simulink model "KitGewerk2_v1_2_Kommunikation_robi"  (R2014a)
settings: Solver=ode3  StartTime=0.0  StopTime=inf  FixedStep=0.005  RelTol=1e-3
undefined symbols (not defined in the file or in its folder): Com1, Com2, none
libraries: slrtlib x14, dspswit3 x3, simulink x2, xpcseriallib x2
(part 1 of 2)
CloseFcn:
  | rtwprivate ssgencode ModelCloseRequest Robotino_Strecke_reall_2009
settings Model: SimulationMode=external  BufferReuse=off  Creator=atlabor  LastModifiedBy=atlabor
settings SolverCC: EnableConcurrentExecution=on
settings DataIOCC: LimitDataPoints=off  SignalLoggingSaveFormat=ModelDataLogs
settings OptimizationCC: BlockReduction=off  OptimizeBlockIOStorage=off  BufferReuse=off  GlobalBufferReuse=off  ExpressionFolding=off  ExpressionDepthLimit=2147483647  LocalBlockOutputs=off  InitFltsAndDblsToZero=on
settings DebuggingCC: SaveWithParameterizedLinksMsg=none  UnderspecifiedInitializationDetection=Classic  FcnCallInpInsideContextMsg=UseLocalSettings  StateNameClashWarn=warning
settings HardwareCC: ProdIntDivRoundTo=Zero  ProdEndianess=LittleEndian  ProdHWDeviceType=Generic->32-bit x86 compatible
settings SFSimCC: SimParseCustomCode=off
settings RTWCC: SystemTargetFile=slrt.tlc  TemplateMakefile=slrt_default_tmf  Description=Simulink Real-Time  ProcessScript=slrt_make_rtw_hook  RTWCompilerOptimization=On
settings SimulinkRealTimeCC: GeneratePreprocessorConditionals=Disable all  EnableShiftOperators=on

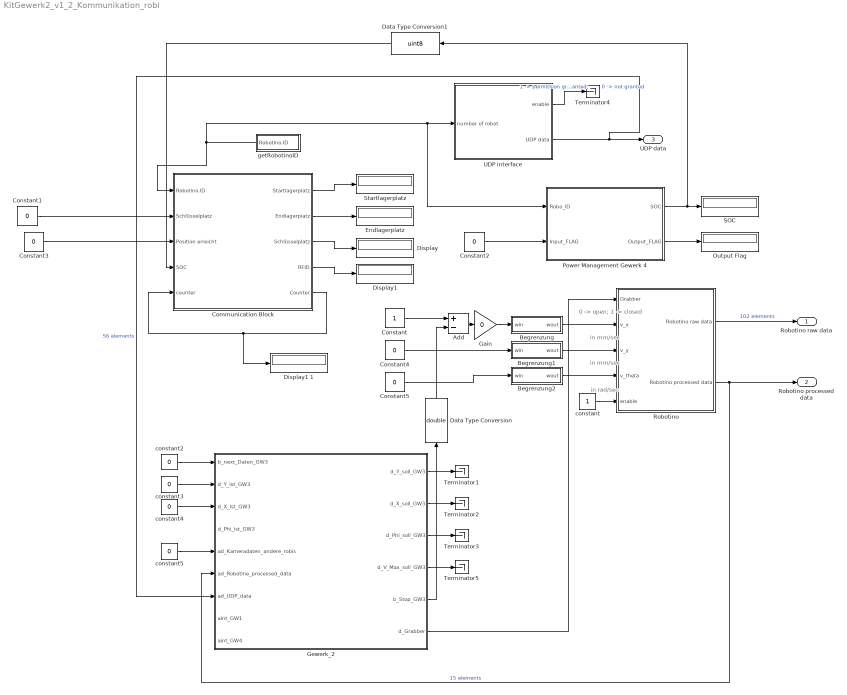
== system KitGewerk2_v1_2_Kommunikation_robi ==
  note: 0 -> open; 1 -> closed
  note: in rad/sec
  note: in mm/sec
  note: in mm/sec
  Add : Sum  Inputs=+-
  Begrenzung : MATLAB Function  TreatAsAtomicUnit=on
  Begrenzung1 : MATLAB Function  TreatAsAtomicUnit=on
  Begrenzung2 : MATLAB Function  TreatAsAtomicUnit=on
  Communication Block : Subsystem
  Constant : Constant
  Constant1 : Constant  Value=0  OutDataTypeStr=boolean
  Constant2 : Constant  Value=0  OutDataTypeStr=uint8
  Constant3 : Constant  Value=0  OutDataTypeStr=boolean
  Constant4 : Constant  Value=0
  Constant5 : Constant  Value=0
  Data Type Conversion : DataTypeConversion  OutDataTypeStr=double
  Data Type Conversion1 : DataTypeConversion  OutDataTypeStr=uint8
  Display : Display
  "Display1 " : Display
  Display1 1 : Display
  Endlagerplatz : Display
  Gain : Gain  Gain=0
  Gewerk_2 : Subsystem
  Output Flag : Display
  Power Management Gewerk 4 : Subsystem
  Robotino : Subsystem
  SOC : Display
  Startlagerplatz : Display
  Terminator{1..5} (5 alike) : Terminator
  UDP interface : Subsystem
  constant : Constant
  constant2 : Constant  Value=0  OutDataTypeStr=boolean
  constant3 : Constant  Value=0  OutDataTypeStr=double
  constant4 : Constant  Value=0
  constant5 : Constant  Value=0
  getRobotinoID : Subsystem
  Robotino raw data : Outport
  Robotino processed data : Outport  Port=2
  UDP data : Outport  Port=3
  wires:
  Robotino/1(Robotino raw data) -> Robotino raw data/1  "102 elements"
  Begrenzung1/1(wout) -> Robotino/3(v_y)
  Begrenzung/1(wout) -> Robotino/2(v_x)
  UDP interface/1(enable) -> Terminator4/1  "1 -> permission granted;        0 -> not granted"
  constant/1 -> Robotino/5(enable)
  getRobotinoID/1(Robotino.ID) -> Power Management Gewerk 4/1(Robo_ID), UDP interface/1(number of robot), Communication Block/1(Robotino.ID)
  Begrenzung2/1(wout) -> Robotino/4(v_theta)
  UDP interface/2(UDP data) -> Gewerk_2/7(ad_UDP_data), UDP data/1  "56 elements"
  Robotino/2(Robotino processed data) -> Gewerk_2/6(ad_Robotine_processed_data), Robotino processed data/1  "15 elements"
  constant3/1 -> Gewerk_2/2(d_Y_ist_GW3)
  constant4/1 -> Gewerk_2/3(d_X_ist_GW3)
  constant5/1 -> Gewerk_2/5(ad_Kameradaten_andere_robis)
  Gewerk_2/1(d_Y_soll_GW3) -> Terminator1/1
  Gewerk_2/2(d_X_soll_GW3) -> Terminator2/1
  Gewerk_2/3(d_Phi_soll_GW3) -> Terminator3/1
  Gewerk_2/4(d_V_Max_soll_GW3) -> Terminator5/1
  Communication Block/1(Startlagerplatz) -> Startlagerplatz/1
  Add/1 -> Gain/1
  Constant/1 -> Add/1
  constant2/1 -> Gewerk_2/1(b_next_Daten_GW3)
  Gain/1 -> Begrenzung/1(win)
  Gewerk_2/5(b_Stop_GW3) -> Data Type Conversion/1
  Gewerk_2/6(d_Grabber) -> Robotino/1(Grabber)
  Data Type Conversion/1 -> Add/2
  Power Management Gewerk 4/1(SOC) -> Data Type Conversion1/1, SOC/1
  Power Management Gewerk 4/2(Output_FLAG) -> Output Flag/1
  Constant2/1 -> Power Management Gewerk 4/2(Input_FLAG)
  Constant1/1 -> Communication Block/2("Schlüsselplatz ")
  Constant3/1 -> Communication Block/3(Position erreicht)
  Communication Block/5(Counter) -> Display1 1/1, Communication Block/5(counter)
  Communication Block/2(Endlagerplatz) -> Endlagerplatz/1
  Constant4/1 -> Begrenzung1/1(win)
  Constant5/1 -> Begrenzung2/1(win)
  Communication Block/3(Schlüsselplatz) -> Display/1
  Communication Block/4(RFID) -> "Display1 "/1
  Data Type Conversion1/1 -> Communication Block/4(SOC)

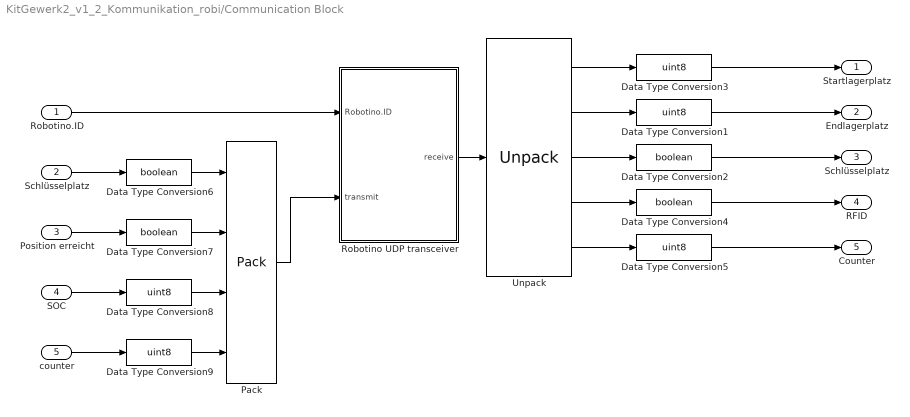
== system KitGewerk2_v1_2_Kommunikation_robi/Communication Block ==
  Robotino.ID : Inport
  "Schlüsselplatz " : Inport  Port=2
  Position erreicht : Inport  Port=3
  SOC : Inport  Port=4
  counter : Inport  Port=5
  Data Type Conversion{1,3,5,8..9} (5 alike) : DataTypeConversion  OutDataTypeStr=uint8
  Data Type Conversion{2,4,6..7} (4 alike) : DataTypeConversion  OutDataTypeStr=boolean
  Pack : slrtlib/UDP/Pack   datatypes={'boolean','boolean','uint8','uint8'}  byteAlign=1
  Robotino UDP transceiver : Subsystem
  Unpack : slrtlib/UDP/Unpack   dimensions={1, 1, 1, 1, 1}  datatypes={'uint8','uint8','boolean','boolean','uint8'}  byteAlign=1
  Startlagerplatz : Outport
  Endlagerplatz : Outport  Port=2
  Schlüsselplatz : Outport  Port=3
  RFID : Outport  Port=4
  Counter : Outport  Port=5
  wires:
  Unpack/1 -> Data Type Conversion3/1
  Unpack/5 -> Data Type Conversion5/1
  Unpack/2 -> Data Type Conversion1/1
  Unpack/3 -> Data Type Conversion2/1
  Unpack/4 -> Data Type Conversion4/1
  Data Type Conversion1/1 -> Endlagerplatz/1
  Data Type Conversion2/1 -> Schlüsselplatz/1
  Data Type Conversion3/1 -> Startlagerplatz/1
  Data Type Conversion4/1 -> RFID/1
  Data Type Conversion5/1 -> Counter/1
  "Schlüsselplatz "/1 -> Data Type Conversion6/1
  Pack/1 -> Robotino UDP transceiver/2(transmit)
  Data Type Conversion6/1 -> Pack/1
  Data Type Conversion7/1 -> Pack/2
  Position erreicht/1 -> Data Type Conversion7/1
  Robotino.ID/1 -> Robotino UDP transceiver/1(Robotino.ID)
  Robotino UDP transceiver/1(receive) -> Unpack/1
  SOC/1 -> Data Type Conversion8/1
  Data Type Conversion8/1 -> Pack/3
  counter/1 -> Data Type Conversion9/1
  Data Type Conversion9/1 -> Pack/4

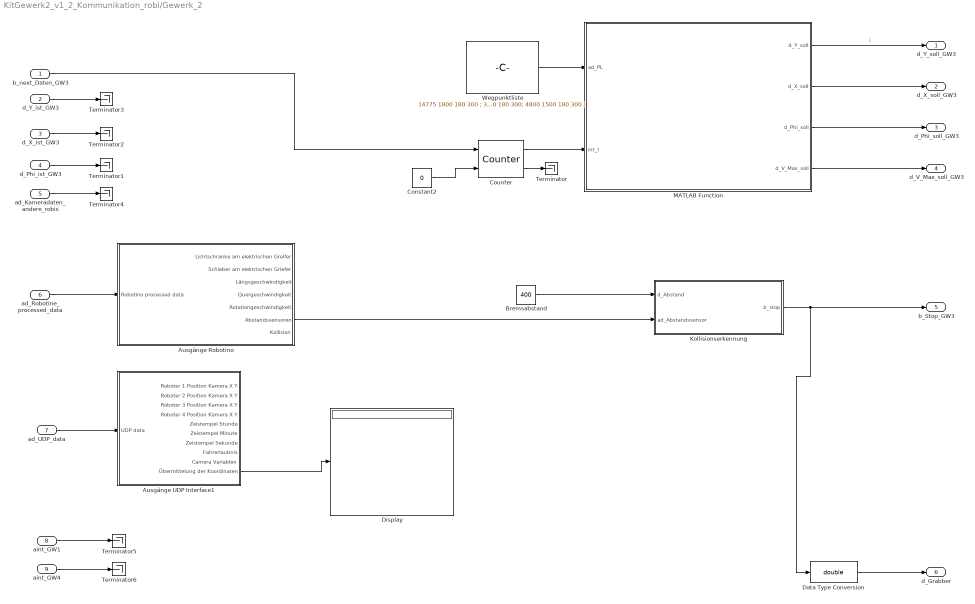
== system KitGewerk2_v1_2_Kommunikation_robi/Gewerk_2 ==
  b_next_Daten_GW3 : Inport  OutDataTypeStr=boolean
  d_Y_ist_GW3 : Inport  Port=2  OutDataTypeStr=double
  d_X_ist_GW3 : Inport  Port=3  OutDataTypeStr=double
  d_Phi_ist_GW3 : Inport  Port=4  OutDataTypeStr=double
  ad_Kameradaten_andere_robis : Inport  Port=5  OutDataTypeStr=double
  ad_Robotine_processed_data : Inport  Port=6
  ad_UDP_data : Inport  Port=7  OutDataTypeStr=double
  aint_GW1 : Inport  Port=8  OutDataTypeStr=boolean
  aint_GW4 : Inport  Port=9  OutDataTypeStr=boolean
  Ausgänge Robotino : Subsystem
  Ausgänge UDP Interface1 : Subsystem
  Bremsabstand : Constant  Value=400  OutDataTypeStr=double
  Constant2 : Constant  Value=0
  Counter : dspswit3/Counter  Direction=Up  CountEvent=Rising edge  CounterSize=User defined  MaxCount=16  InitialCount=0  Output=Count and Hit  HitValue=16  ResetInput=on  SamplesPerFrame=1  Ts=1  CntDtype=int32  HitDtype=Logical
  Data Type Conversion : DataTypeConversion  OutDataTypeStr=double
  Display : Display
  Kollisionserkennung : MATLAB Function  TreatAsAtomicUnit=on
  MATLAB Function : MATLAB Function  TreatAsAtomicUnit=on
  Terminator{,1..6} (7 alike) : Terminator
  Wegpunktliste : Constant  Value=[4775 1800 180 300 ; 3745 1800 180 300; 2540 2100 180 300; 2160 2100 180 300; 1678 1894 180 300; 1373 1846 180 300; 1155 1627 180 300; 1106 1321 180 300; 1246 1046 180 300; 1522 906 180 300; 1827 954 180 300; 2300 954 180 300; 2800 1500 180 300; 3300 1000 180 300; 3800 1500 180 300; 4300 1000 180 300; 4800 1500 180 300 ]  OutDataTypeStr=double
  d_Y_soll_GW3 : Outport  OutDataTypeStr=double
  d_X_soll_GW3 : Outport  Port=2  OutDataTypeStr=double
  d_Phi_soll_GW3 : Outport  Port=3  OutDataTypeStr=double
  d_V_Max_soll_GW3 : Outport  Port=4  OutDataTypeStr=double
  b_Stop_GW3 : Outport  Port=5  OutDataTypeStr=boolean
  d_Grabber : Outport  Port=6  OutDataTypeStr=double
  wires:
  d_Y_ist_GW3/1 -> Terminator3/1
  ad_Kameradaten_andere_robis/1 -> Terminator4/1
  d_Phi_ist_GW3/1 -> Terminator1/1
  d_X_ist_GW3/1 -> Terminator2/1
  Wegpunktliste/1 -> MATLAB Function/1(ad_PL)
  Counter/1 -> MATLAB Function/2(int_I)
  MATLAB Function/2(d_X_soll) -> d_X_soll_GW3/1
  b_next_Daten_GW3/1 -> Counter/1
  MATLAB Function/1(d_Y_soll) -> d_Y_soll_GW3/1  "i"
  MATLAB Function/4(d_V_Max_soll) -> d_V_Max_soll_GW3/1
  MATLAB Function/3(d_Phi_soll) -> d_Phi_soll_GW3/1
  Constant2/1 -> Counter/2
  Counter/2 -> Terminator/1
  Kollisionserkennung/1(b_stop) -> Data Type Conversion/1, b_Stop_GW3/1
  Ausgänge Robotino/6(Abstandssensoren) -> Kollisionserkennung/2(ad_Abstandssensor)
  Bremsabstand/1 -> Kollisionserkennung/1(d_Abstand)
  ad_Robotine_processed_data/1 -> Ausgänge Robotino/1(Robotino processed data)
  ad_UDP_data/1 -> Ausgänge UDP Interface1/1(UDP data)
  Data Type Conversion/1 -> d_Grabber/1
  aint_GW4/1 -> Terminator6/1
  aint_GW1/1 -> Terminator5/1
  Ausgänge UDP Interface1/10(Übermittelung der Koordinaten) -> Display/1

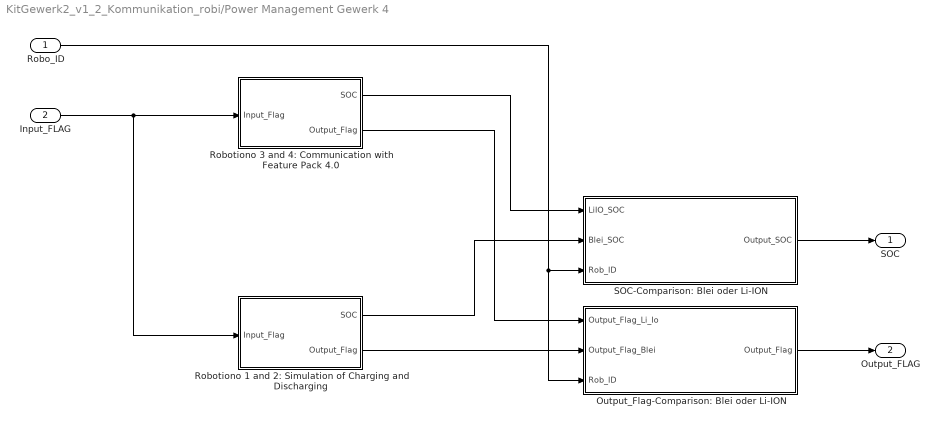
== system KitGewerk2_v1_2_Kommunikation_robi/Power Management Gewerk 4 ==
  Robo_ID : Inport
  Input_FLAG : Inport  Port=2
  Output_Flag-Comparison: Blei oder Li-ION : MATLAB Function  TreatAsAtomicUnit=on
  Robotiono 1 and 2: Simulation of Charging and Discharging : Subsystem
  Robotiono 3 and 4: Communication with Feature Pack 4.0 : Subsystem
  SOC-Comparison: Blei oder Li-ION : MATLAB Function  TreatAsAtomicUnit=on
  SOC : Outport
  Output_FLAG : Outport  Port=2
  wires:
  Output_Flag-Comparison: Blei oder Li-ION/1(Output_Flag) -> Output_FLAG/1
  Robo_ID/1 -> Output_Flag-Comparison: Blei oder Li-ION/3(Rob_ID), SOC-Comparison: Blei oder Li-ION/3(Rob_ID)
  Robotiono 3 and 4: Communication with Feature Pack 4.0/1(SOC) -> SOC-Comparison: Blei oder Li-ION/1(LiIO_SOC)
  SOC-Comparison: Blei oder Li-ION/1(Output_SOC) -> SOC/1
  Input_FLAG/1 -> Robotiono 1 and 2: Simulation of Charging and Discharging/1(Input_Flag), Robotiono 3 and 4: Communication with Feature Pack 4.0/1(Input_Flag)
  Robotiono 1 and 2: Simulation of Charging and Discharging/1(SOC) -> SOC-Comparison: Blei oder Li-ION/2(Blei_SOC)
  Robotiono 1 and 2: Simulation of Charging and Discharging/2(Output_Flag) -> Output_Flag-Comparison: Blei oder Li-ION/2(Output_Flag_Blei)
  Robotiono 3 and 4: Communication with Feature Pack 4.0/2(Output_Flag) -> Output_Flag-Comparison: Blei oder Li-ION/1(Output_Flag_Li_Io)

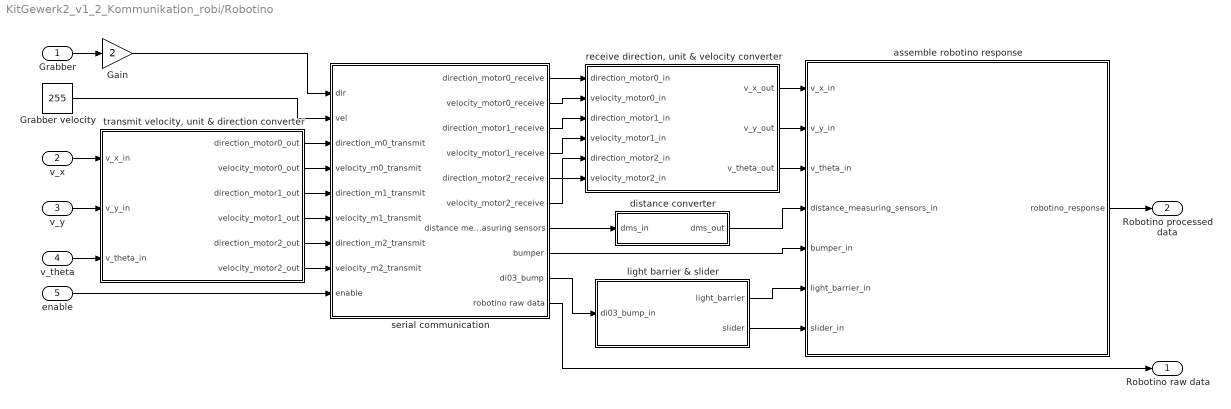
== system KitGewerk2_v1_2_Kommunikation_robi/Robotino ==
  Grabber : Inport
  v_x : Inport  Port=2
  v_y : Inport  Port=3
  v_theta : Inport  Port=4
  enable : Inport  Port=5
  Gain : Gain  Gain=2
  Grabber velocity : Constant  Value=255
  assemble robotino response : MATLAB Function  TreatAsAtomicUnit=on
  distance converter : MATLAB Function  TreatAsAtomicUnit=on
  light barrier & slider : MATLAB Function  TreatAsAtomicUnit=on
  "receive direction, unit & velocity converter" : MATLAB Function  TreatAsAtomicUnit=on
  serial communication : Subsystem
  "transmit velocity, unit & direction converter" : MATLAB Function  TreatAsAtomicUnit=on
  Robotino raw data : Outport
  Robotino processed data : Outport  Port=2
  wires:
  "transmit velocity, unit & direction converter"/1(direction_motor0_out) -> serial communication/3(direction_m0_transmit)
  "transmit velocity, unit & direction converter"/2(velocity_motor0_out) -> serial communication/4(velocity_m0_transmit)
  "transmit velocity, unit & direction converter"/3(direction_motor1_out) -> serial communication/5(direction_m1_transmit)
  "transmit velocity, unit & direction converter"/4(velocity_motor1_out) -> serial communication/6(velocity_m1_transmit)
  "transmit velocity, unit & direction converter"/5(direction_motor2_out) -> serial communication/7(direction_m2_transmit)
  "transmit velocity, unit & direction converter"/6(velocity_motor2_out) -> serial communication/8(velocity_m2_transmit)
  v_x/1 -> "transmit velocity, unit & direction converter"/1(v_x_in)
  v_y/1 -> "transmit velocity, unit & direction converter"/2(v_y_in)
  v_theta/1 -> "transmit velocity, unit & direction converter"/3(v_theta_in)
  "receive direction, unit & velocity converter"/2(v_y_out) -> assemble robotino response/2(v_y_in)
  enable/1 -> serial communication/9(enable)
  serial communication/1(direction_motor0_receive) -> "receive direction, unit & velocity converter"/1(direction_motor0_in)
  serial communication/7(distance measuring sensors) -> distance converter/1(dms_in)
  serial communication/10(robotino raw data) -> Robotino raw data/1
  serial communication/9(di03_bump) -> light barrier & slider/1(di03_bump_in)
  "receive direction, unit & velocity converter"/1(v_x_out) -> assemble robotino response/1(v_x_in)
  "receive direction, unit & velocity converter"/3(v_theta_out) -> assemble robotino response/3(v_theta_in)
  assemble robotino response/1(robotino_response) -> Robotino processed data/1
  Grabber/1 -> Gain/1
  Gain/1 -> serial communication/1(dir)
  distance converter/1(dms_out) -> assemble robotino response/4(distance_measuring_sensors_in)
  light barrier & slider/2(slider) -> assemble robotino response/7(slider_in)
  light barrier & slider/1(light_barrier) -> assemble robotino response/6(light_barrier_in)
  serial communication/8(bumper) -> assemble robotino response/5(bumper_in)
  serial communication/2(velocity_motor0_receive) -> "receive direction, unit & velocity converter"/2(velocity_motor0_in)
  serial communication/3(direction_motor1_receive) -> "receive direction, unit & velocity converter"/3(direction_motor1_in)
  serial communication/4(velocity_motor1_receive) -> "receive direction, unit & velocity converter"/4(velocity_motor1_in)
  serial communication/5(direction_motor2_receive) -> "receive direction, unit & velocity converter"/5(direction_motor2_in)
  serial communication/6(velocity_motor2_receive) -> "receive direction, unit & velocity converter"/6(velocity_motor2_in)
  Grabber velocity/1 -> serial communication/2(vel)

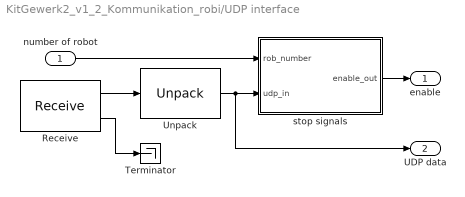
== system KitGewerk2_v1_2_Kommunikation_robi/UDP interface ==
  number of robot : Inport
  Receive : slrtlib/UDP/Receive   ipAddress=0.0.0.0  ipPort=25000  width=448  vblLen=off  sampletime=-1
  Terminator : Terminator
  Unpack : slrtlib/UDP/Unpack   dimensions={[56]}  datatypes={'double'}  byteAlign=1
  stop signals : MATLAB Function  TreatAsAtomicUnit=on
  enable : Outport
  UDP data : Outport  Port=2
  wires:
  Unpack/1 -> stop signals/2(udp_in), UDP data/1
  Receive/1 -> Unpack/1
  Receive/2 -> Terminator/1
  stop signals/1(enable_out) -> enable/1
  number of robot/1 -> stop signals/1(rob_number)

== system KitGewerk2_v1_2_Kommunikation_robi/getRobotinoID ==
  note: Executing only once at start after 10ms
  Step : Step  Time=0.01  SampleTime=0
  getIDfromFlash : Subsystem
  Robotino.ID : Outport
  wires:
  Step/1 -> getIDfromFlash/Trigger
  getIDfromFlash/1(RobotinoID) -> Robotino.ID/1

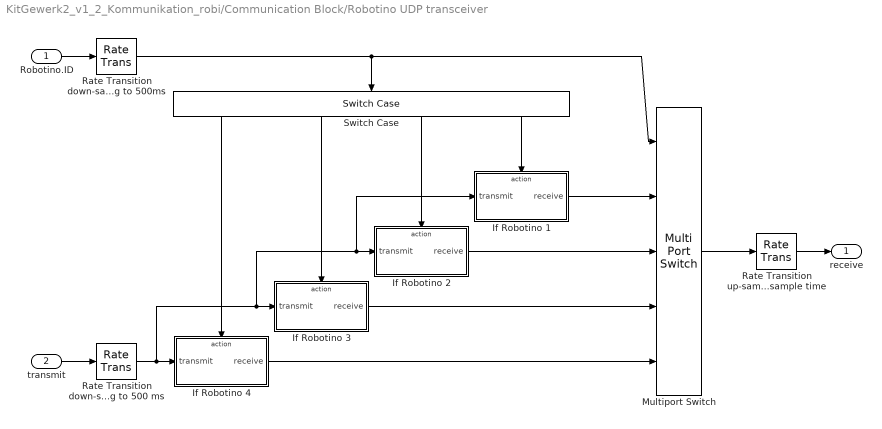
== system KitGewerk2_v1_2_Kommunikation_robi/Communication Block/Robotino UDP transceiver ==
  Robotino.ID : Inport
  transmit : Inport  Port=2
  If Robotino 1 : Subsystem  TreatAsAtomicUnit=on
  If Robotino 2 : Subsystem  TreatAsAtomicUnit=on
  If Robotino 3 : Subsystem  TreatAsAtomicUnit=on
  If Robotino 4 : Subsystem  TreatAsAtomicUnit=on
  Multiport Switch : MultiPortSwitch  Inputs=4
  Rate Transition down-sampling to 500 ms : RateTransition  OutPortSampleTime=0.5
  Rate Transition down-sampling to 500ms : RateTransition  OutPortSampleTime=0.5
  Rate Transition up-sampling to fundamental sample time : RateTransition
  Switch Case : SwitchCase  CaseConditions={4,3,2,1}  ShowDefaultCase=off
  receive : Outport
  wires:
  Switch Case/1 -> If Robotino 4/Action
  Switch Case/2 -> If Robotino 3/Action
  Switch Case/3 -> If Robotino 2/Action
  Switch Case/4 -> If Robotino 1/Action
  Multiport Switch/1 -> Rate Transition up-sampling to fundamental sample time/1
  If Robotino 1/1(receive) -> Multiport Switch/2
  If Robotino 3/1(receive) -> Multiport Switch/4
  If Robotino 2/1(receive) -> Multiport Switch/3
  If Robotino 4/1(receive) -> Multiport Switch/5
  transmit/1 -> Rate Transition down-sampling to 500 ms/1
  Rate Transition up-sampling to fundamental sample time/1 -> receive/1
  Rate Transition down-sampling to 500 ms/1 -> If Robotino 4/1(transmit), If Robotino 3/1(transmit), If Robotino 2/1(transmit), If Robotino 1/1(transmit)
  Robotino.ID/1 -> Rate Transition down-sampling to 500ms/1
  Rate Transition down-sampling to 500ms/1 -> Switch Case/1, Multiport Switch/1

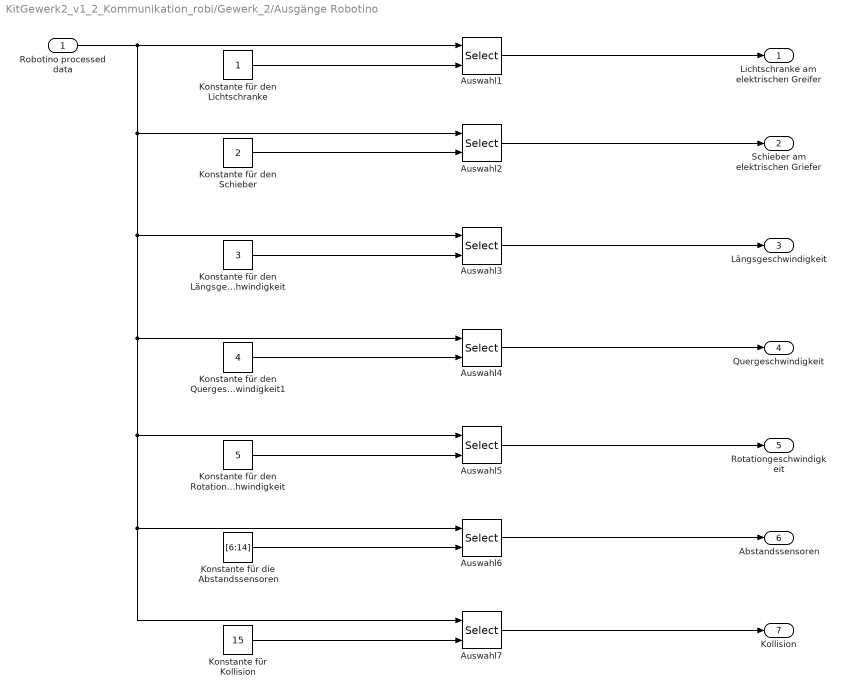
== system KitGewerk2_v1_2_Kommunikation_robi/Gewerk_2/Ausgänge Robotino ==
  Robotino processed data : Inport
  Auswahl{1..7} (7 alike) : Selector  InputPortWidth=15  IndexOptions=Index vector (port)  Indices=[1 3]
  "Konstante für Kollision " : Constant  Value=15
  Konstante für den Lichtschranke : Constant
  Konstante für den Längsgeschwindigkeit : Constant  Value=3
  Konstante für den Quergeschwindigkeit1 : Constant  Value=4
  Konstante für den Rotationegeschwindigkeit : Constant  Value=5
  Konstante für den Schieber : Constant  Value=2
  Konstante für die Abstandssensoren : Constant  Value=[6:14]
  Lichtschranke am elektrischen Greifer : Outport
  "Schieber am elektrischen Griefer " : Outport  Port=2
  "Längsgeschwindigkeit " : Outport  Port=3
  Quergeschwindigkeit : Outport  Port=4
  "Rotationgeschwindigkeit " : Outport  Port=5
  Abstandssensoren : Outport  Port=6
  Kollision : Outport  Port=7
  wires:
  Auswahl1/1 -> Lichtschranke am elektrischen Greifer/1
  Robotino processed data/1 -> Auswahl1/1, Auswahl5/1, Auswahl7/1, Auswahl6/1, Auswahl4/1, Auswahl3/1, Auswahl2/1
  Konstante für den Lichtschranke/1 -> Auswahl1/2
  Konstante für den Schieber/1 -> Auswahl2/2
  Auswahl2/1 -> "Schieber am elektrischen Griefer "/1
  Konstante für den Längsgeschwindigkeit/1 -> Auswahl3/2
  Auswahl3/1 -> "Längsgeschwindigkeit "/1
  Konstante für den Quergeschwindigkeit1/1 -> Auswahl4/2
  Auswahl4/1 -> Quergeschwindigkeit/1
  Auswahl5/1 -> "Rotationgeschwindigkeit "/1
  Konstante für den Rotationegeschwindigkeit/1 -> Auswahl5/2
  Konstante für die Abstandssensoren/1 -> Auswahl6/2
  Auswahl6/1 -> Abstandssensoren/1
  Auswahl7/1 -> Kollision/1
  "Konstante für Kollision "/1 -> Auswahl7/2

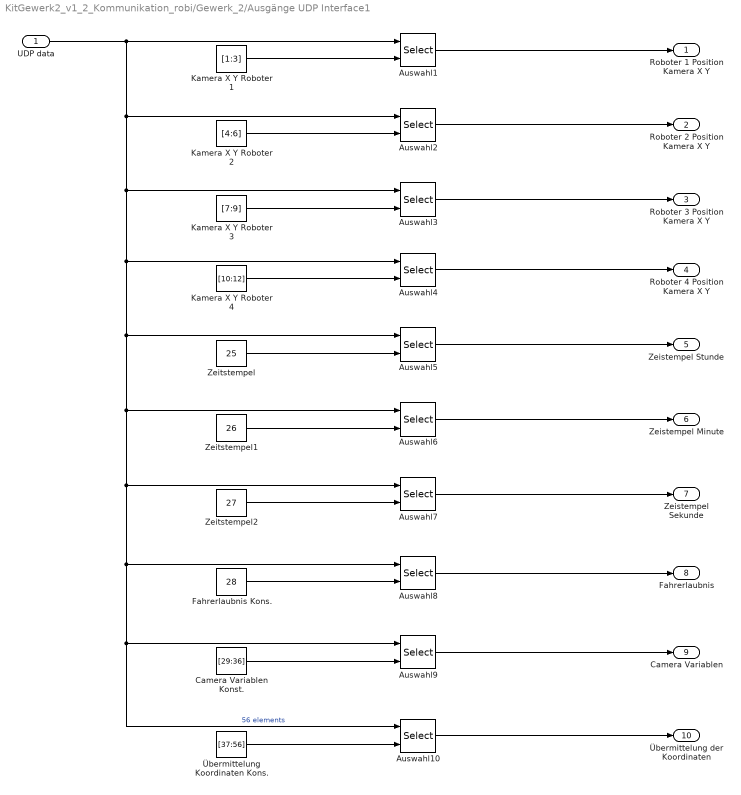
== system KitGewerk2_v1_2_Kommunikation_robi/Gewerk_2/Ausgänge UDP Interface1 ==
  UDP data : Inport
  Auswahl{1..10} (10 alike) : Selector  InputPortWidth=56  IndexOptions=Index vector (port)  Indices=[1 3]
  Camera Variablen Konst. : Constant  Value=[29:36]
  Fahrerlaubnis Kons. : Constant  Value=28
  Kamera X Y Roboter 1 : Constant  Value=[1:3]
  Kamera X Y Roboter 2 : Constant  Value=[4:6]
  Kamera X Y Roboter 3 : Constant  Value=[7:9]
  Kamera X Y Roboter 4 : Constant  Value=[10:12]
  Zeitstempel : Constant  Value=25
  Zeitstempel1 : Constant  Value=26
  Zeitstempel2 : Constant  Value=27
  Übermittelung Koordinaten Kons. : Constant  Value=[37:56]
  Roboter 1 Position Kamera X Y : Outport
  Roboter 2 Position Kamera X Y : Outport  Port=2
  Roboter 3 Position Kamera X Y : Outport  Port=3
  Roboter 4 Position Kamera X Y : Outport  Port=4
  Zeistempel Stunde : Outport  Port=5
  Zeistempel Minute : Outport  Port=6
  Zeistempel Sekunde : Outport  Port=7
  Fahrerlaubnis : Outport  Port=8
  Camera Variablen : Outport  Port=9
  Übermittelung der Koordinaten : Outport  Port=10
  wires:
  Kamera X Y Roboter 1/1 -> Auswahl1/2
  Kamera X Y Roboter 2/1 -> Auswahl2/2
  Kamera X Y Roboter 3/1 -> Auswahl3/2
  Kamera X Y Roboter 4/1 -> Auswahl4/2
  Auswahl1/1 -> Roboter 1 Position Kamera X Y/1
  Auswahl3/1 -> Roboter 3 Position Kamera X Y/1
  Auswahl2/1 -> Roboter 2 Position Kamera X Y/1
  Auswahl4/1 -> Roboter 4 Position Kamera X Y/1
  Zeitstempel/1 -> Auswahl5/2
  Auswahl5/1 -> Zeistempel Stunde/1
  Zeitstempel1/1 -> Auswahl6/2
  Auswahl6/1 -> Zeistempel Minute/1
  Zeitstempel2/1 -> Auswahl7/2
  Auswahl7/1 -> Zeistempel Sekunde/1
  Fahrerlaubnis Kons./1 -> Auswahl8/2
  Auswahl8/1 -> Fahrerlaubnis/1
  Camera Variablen Konst./1 -> Auswahl9/2
  Auswahl9/1 -> Camera Variablen/1
  UDP data/1 -> Auswahl2/1, Auswahl10/1, Auswahl9/1, Auswahl8/1, Auswahl7/1, Auswahl6/1, Auswahl5/1, Auswahl4/1, Auswahl3/1, Auswahl1/1  "56 elements"
  Übermittelung Koordinaten Kons./1 -> Auswahl10/2
  Auswahl10/1 -> Übermittelung der Koordinaten/1

== system KitGewerk2_v1_2_Kommunikation_robi/Power Management Gewerk 4/Robotiono 1 and 2: Simulation of Charging and Discharging ==
  Input_Flag : Inport
  Simulation of Charging and Discharging : Subsystem
  SOC : Outport
  Output_Flag : Outport  Port=2
  wires:
  Simulation of Charging and Discharging/2(Output_Flag) -> Output_Flag/1
  Input_Flag/1 -> Simulation of Charging and Discharging/1(Input_Flag)
  Simulation of Charging and Discharging/1(SOC) -> SOC/1

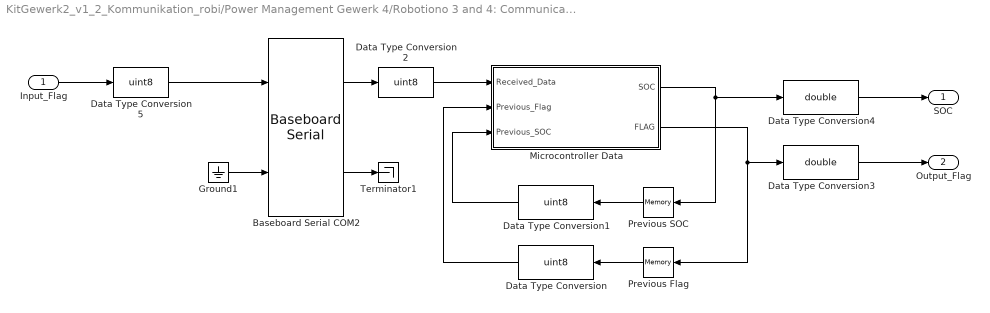
== system KitGewerk2_v1_2_Kommunikation_robi/Power Management Gewerk 4/Robotiono 3 and 4: Communication with Feature Pack 4.0 ==
  Input_Flag : Inport
  Baseboard Serial COM2 : xpcseriallib/Mainboard/Baseboard Serial  group=Receive Setup  port=1  irqnum=3  saddr1=0x2F8  saddr2=0x2E8  config=Com2/none  baud1=9600  parity1=None  ndata1=8  nstop1=1  fifomode1=16 deep  rlevel1=1  automode1=off  xmtfifosize1=10240  xmtdatatype1=8 bit uint null terminated  rcvfifosize1=10240  rcvmaxread1=3  rcvminread1=1  rcvusedelim1=on  rcvdelim1=10  rcvdatatype1=count+16 bit uint  rcvsampletime1=-1  baud2=1200  parity2=None  ndata2=8  nstop2=1  fifomode2=16 deep  rlevel2=1  automode2=off  xmtfifosize2=1024  xmtdatatype2=8 bit uint null terminated  rcvfifosize2=1024  rcvmaxread2=101  rcvminread2=1  rcvusedelim2=on  rcvdelim2=10  rcvdatatype2=8 bit uint null terminated  rcvsampletime2=-1
      link override FIFO read 1: maxsize=101  minsize=1  usedelimiter=on  delimiter=99  outputtype=count+16 bit uint  sampletime=dt / 2
      link override FIFO read 2: maxsize=101  minsize=1  usedelimiter=on  delimiter=99  outputtype=count+16 bit uint  sampletime=dt / 2
      link override FIFO write 1: size=1024  inputtype=8 bit int null terminated  sampletime=-1  id=XMT channel 1, IRQ 4
      link override FIFO write 2: size=1024  inputtype=8 bit uint null terminated  id=XMT channel 2, IRQ 4
      link override IRQ Source: irqNo=Auto (PCI only)
      link override Setup1: baud=115200  width=8  nstop=1  parity=None  fmode=16 deep  rlevel=half full  ctsmode=off
      link override Setup2: baud=4800  width=8  nstop=1  parity=None  fmode=16 deep  rlevel=half full  ctsmode=off
  Data Type Conversion{,1..2,5} (4 alike) : DataTypeConversion  OutDataTypeStr=uint8
  Data Type Conversion3 : DataTypeConversion  OutDataTypeStr=double
  Data Type Conversion4 : DataTypeConversion  OutDataTypeStr=double
  Ground1 : Ground
  Microcontroller Data : MATLAB Function  TreatAsAtomicUnit=on
  Previous Flag : Memory
  Previous SOC : Memory
  Terminator1 : Terminator
  SOC : Outport
  Output_Flag : Outport  Port=2
  wires:
  Baseboard Serial COM2/2 -> Terminator1/1
  Ground1/1 -> Baseboard Serial COM2/2
  Baseboard Serial COM2/1 -> Data Type Conversion2/1
  Microcontroller Data/2(FLAG) -> Previous Flag/1, Data Type Conversion3/1
  Microcontroller Data/1(SOC) -> Previous SOC/1, Data Type Conversion4/1
  Input_Flag/1 -> Data Type Conversion5/1
  Previous SOC/1 -> Data Type Conversion1/1
  Previous Flag/1 -> Data Type Conversion/1
  Data Type Conversion/1 -> Microcontroller Data/2(Previous_Flag)
  Data Type Conversion1/1 -> Microcontroller Data/3(Previous_SOC)
  Data Type Conversion2/1 -> Microcontroller Data/1(Received_Data)
  Data Type Conversion3/1 -> Output_Flag/1
  Data Type Conversion4/1 -> SOC/1
  Data Type Conversion5/1 -> Baseboard Serial COM2/1

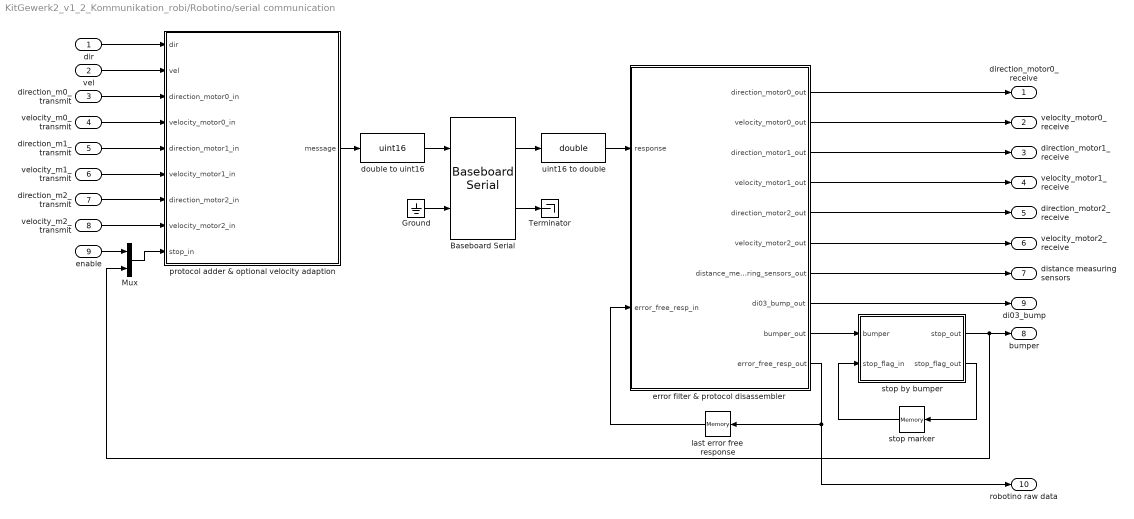
== system KitGewerk2_v1_2_Kommunikation_robi/Robotino/serial communication ==
  dir : Inport
  vel : Inport  Port=2
  direction_m0_transmit : Inport  Port=3
  velocity_m0_transmit : Inport  Port=4
  direction_m1_transmit : Inport  Port=5
  velocity_m1_transmit : Inport  Port=6
  direction_m2_transmit : Inport  Port=7
  velocity_m2_transmit : Inport  Port=8
  enable : Inport  Port=9
  Baseboard Serial : xpcseriallib/Mainboard/Baseboard Serial  group=Transmit Setup  port=2  irqnum=4  saddr1=0x3f8  saddr2=0x3e8  config=Com1/none  baud1=115200  parity1=None  ndata1=8  nstop1=1  fifomode1=16 deep  rlevel1=almost full  automode1=off  xmtfifosize1=10240  xmtdatatype1=count+16 bit uint  rcvfifosize1=10240  rcvmaxread1=101  rcvminread1=1  rcvusedelim1=on  rcvdelim1=99  rcvdatatype1=count+16 bit uint  rcvsampletime1=-1  baud2=115200  parity2=None  ndata2=8  nstop2=1  fifomode2=16 deep  rlevel2=almost full  automode2=off  xmtfifosize2=10240  xmtdatatype2=count+16 bit uint  rcvfifosize2=10240  rcvmaxread2=101  rcvminread2=1  rcvusedelim2=on  rcvdelim2=99  rcvdatatype2=count+16 bit uint  rcvsampletime2=-1
      link override FIFO read 1: maxsize=101  minsize=1  usedelimiter=on  delimiter=99  outputtype=count+16 bit uint  sampletime=dt / 2
      link override FIFO read 2: maxsize=101  minsize=1  usedelimiter=on  delimiter=99  outputtype=count+16 bit uint  sampletime=dt / 2
      link override FIFO write 1: size=1024  inputtype=count+16 bit uint  sampletime=-1  id=XMT channel 1, IRQ 4
      link override FIFO write 2: size=1024  inputtype=8 bit uint null terminated  id=XMT channel 2, IRQ 4
      link override Setup1: baud=115200  width=8  nstop=1  parity=None  fmode=16 deep  rlevel=half full  ctsmode=off
      link override Setup2: baud=4800  width=8  nstop=1  parity=None  fmode=16 deep  rlevel=half full  ctsmode=off
  Ground : Ground
  Mux : Mux  Inputs=2
  Terminator : Terminator
  double to uint16 : DataTypeConversion  OutDataTypeStr=uint16  RndMeth=Nearest
  error filter & protocol disassembler : MATLAB Function  TreatAsAtomicUnit=on
  last error free response : Memory  X0=[zeros(1,102)]
  protocol adder & optional velocity adaption : MATLAB Function  TreatAsAtomicUnit=on
  stop by bumper : MATLAB Function  TreatAsAtomicUnit=on
  stop marker : Memory  X0=[zeros(1,3)]
  uint16 to double : DataTypeConversion  OutDataTypeStr=double  RndMeth=Nearest
  direction_motor0_receive : Outport
  velocity_motor0_receive : Outport  Port=2
  direction_motor1_receive : Outport  Port=3
  velocity_motor1_receive : Outport  Port=4
  direction_motor2_receive : Outport  Port=5
  velocity_motor2_receive : Outport  Port=6
  distance measuring sensors : Outport  Port=7
  bumper : Outport  Port=8
  di03_bump : Outport  Port=9
  robotino raw data : Outport  Port=10
  wires:
  Ground/1 -> Baseboard Serial/2
  Baseboard Serial/2 -> Terminator/1
  double to uint16/1 -> Baseboard Serial/1
  protocol adder & optional velocity adaption/1(message) -> double to uint16/1
  stop marker/1 -> stop by bumper/2(stop_flag_in)
  stop by bumper/2(stop_flag_out) -> stop marker/1
  last error free response/1 -> error filter & protocol disassembler/2(error_free_resp_in)
  error filter & protocol disassembler/10(error_free_resp_out) -> last error free response/1, robotino raw data/1
  error filter & protocol disassembler/1(direction_motor0_out) -> direction_motor0_receive/1
  error filter & protocol disassembler/2(velocity_motor0_out) -> velocity_motor0_receive/1
  error filter & protocol disassembler/3(direction_motor1_out) -> direction_motor1_receive/1
  error filter & protocol disassembler/4(velocity_motor1_out) -> velocity_motor1_receive/1
  direction_m0_transmit/1 -> protocol adder & optional velocity adaption/3(direction_motor0_in)
  error filter & protocol disassembler/5(direction_motor2_out) -> direction_motor2_receive/1
  velocity_m0_transmit/1 -> protocol adder & optional velocity adaption/4(velocity_motor0_in)
  error filter & protocol disassembler/6(velocity_motor2_out) -> velocity_motor2_receive/1
  direction_m1_transmit/1 -> protocol adder & optional velocity adaption/5(direction_motor1_in)
  velocity_m1_transmit/1 -> protocol adder & optional velocity adaption/6(velocity_motor1_in)
  direction_m2_transmit/1 -> protocol adder & optional velocity adaption/7(direction_motor2_in)
  velocity_m2_transmit/1 -> protocol adder & optional velocity adaption/8(velocity_motor2_in)
  error filter & protocol disassembler/9(bumper_out) -> stop by bumper/1(bumper)
  stop by bumper/1(stop_out) -> bumper/1, Mux/2
  error filter & protocol disassembler/7(distance_measuring_sensors_out) -> distance measuring sensors/1
  Baseboard Serial/1 -> uint16 to double/1
  uint16 to double/1 -> error filter & protocol disassembler/1(response)
  enable/1 -> Mux/1
  dir/1 -> protocol adder & optional velocity adaption/1(dir)
  vel/1 -> protocol adder & optional velocity adaption/2(vel)
  Mux/1 -> protocol adder & optional velocity adaption/9(stop_in)
  error filter & protocol disassembler/8(di03_bump_out) -> di03_bump/1

== system KitGewerk2_v1_2_Kommunikation_robi/getRobotinoID/getIDfromFlash ==
  Trigger : TriggerPort
  From File : slrtlib/Target Management/From File   filename='robotino.id'  dataSize=8  bufSize=2000  readSize=512  EOFOption=Seek to beginning  sampTime=-1  show2ports=off
  Unpack : slrtlib/UDP/Unpack   dimensions={[1]}  datatypes={'double'}  byteAlign=1
  RobotinoID : Outport
  wires:
  From File/1 -> Unpack/1
  Unpack/1 -> RobotinoID/1

== system KitGewerk2_v1_2_Kommunikation_robi/Communication Block/Robotino UDP transceiver/If Robotino 1 ==
  transmit : Inport
  Action Port : ActionPort  ActionType=case
  Receive from all : slrtlib/UDP/Receive   ipAddress=0.0.0.0  ipPort=25011  width=5  vblLen=off  sampletime=-1
  Send to all : slrtlib/UDP/Send   ipAddress=255.255.255.255  ipPort=25010  localPort=-1  vblLen=off  sampletime=-1
  Terminator : Terminator
  receive : Outport
  wires:
  Receive from all/1 -> receive/1
  Receive from all/2 -> Terminator/1
  transmit/1 -> Send to all/1

== system KitGewerk2_v1_2_Kommunikation_robi/Communication Block/Robotino UDP transceiver/If Robotino 2 ==
  transmit : Inport
  Action Port : ActionPort  ActionType=case
  Receive from all : slrtlib/UDP/Receive   ipAddress=0.0.0.0  ipPort=25012  width=5  vblLen=off  sampletime=-1
  Send to all : slrtlib/UDP/Send   ipAddress=255.255.255.255  ipPort=25020  localPort=-1  vblLen=off  sampletime=-1
  Terminator : Terminator
  receive : Outport
  wires:
  Receive from all/1 -> receive/1
  Receive from all/2 -> Terminator/1
  transmit/1 -> Send to all/1

== system KitGewerk2_v1_2_Kommunikation_robi/Communication Block/Robotino UDP transceiver/If Robotino 3 ==
  transmit : Inport
  Action Port : ActionPort  ActionType=case
  Receive from all : slrtlib/UDP/Receive   ipAddress=0.0.0.0  ipPort=25013  width=5  vblLen=off  sampletime=-1
  Send to all : slrtlib/UDP/Send   ipAddress=255.255.255.255  ipPort=25030  localPort=-1  vblLen=off  sampletime=-1
  Terminator : Terminator
  receive : Outport
  wires:
  Receive from all/1 -> receive/1
  Receive from all/2 -> Terminator/1
  transmit/1 -> Send to all/1

== system KitGewerk2_v1_2_Kommunikation_robi/Communication Block/Robotino UDP transceiver/If Robotino 4 ==
  transmit : Inport
  Action Port : ActionPort  ActionType=case
  Receive from all : slrtlib/UDP/Receive   ipAddress=0.0.0.0  ipPort=25014  width=5  vblLen=off  sampletime=-1
  Send to all : slrtlib/UDP/Send   ipAddress=255.255.255.255  ipPort=25040  localPort=-1  vblLen=off  sampletime=-1
  Terminator : Terminator
  receive : Outport
  wires:
  Receive from all/1 -> receive/1
  Receive from all/2 -> Terminator/1
  transmit/1 -> Send to all/1

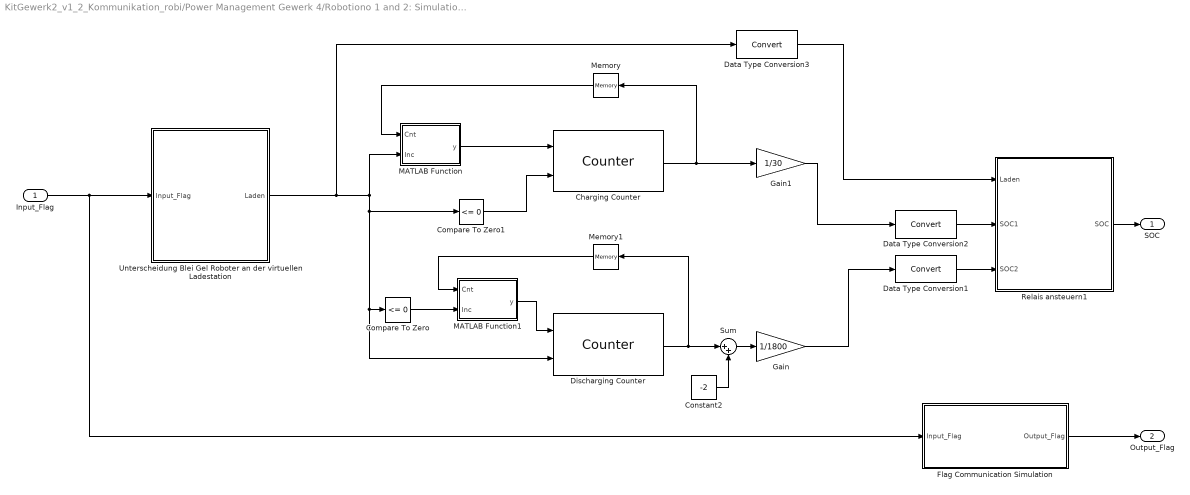
== system KitGewerk2_v1_2_Kommunikation_robi/Power Management Gewerk 4/Robotiono 1 and 2: Simulation of Charging and Discharging/Simulation of Charging and Discharging ==
  Input_Flag : Inport
  Charging Counter : dspswit3/Counter  Direction=Up  CountEvent=Non-zero sample  CounterSize=User defined  MaxCount=3002  InitialCount=0  Output=Count  HitValue=32  ResetInput=on  SamplesPerFrame=1  Ts=1  CntDtype=uint16  HitDtype=Logical
  Compare To Zero : simulink/Logic and Bit Operations/Compare To Zero  relop=<=  OutDataTypeStr=uint8
  Compare To Zero1 : simulink/Logic and Bit Operations/Compare To Zero  relop=<=  OutDataTypeStr=boolean
  Constant2 : Constant  Value=-2
  Data Type Conversion1 : DataTypeConversion
  Data Type Conversion2 : DataTypeConversion
  Data Type Conversion3 : DataTypeConversion
  Discharging Counter : dspswit3/Counter  Direction=Down  CountEvent=Non-zero sample  CounterSize=User defined  MaxCount=180002  InitialCount=180002  Output=Count  HitValue=32  ResetInput=on  SamplesPerFrame=1  Ts=1  CntDtype=uint32  HitDtype=Logical
  Flag Communication Simulation : MATLAB Function  TreatAsAtomicUnit=on
  Gain : Gain  Gain=1/1800
  Gain1 : Gain  Gain=1/30
  MATLAB Function : MATLAB Function  TreatAsAtomicUnit=on
  MATLAB Function1 : MATLAB Function  TreatAsAtomicUnit=on
  Memory : Memory  InheritSampleTime=on
  Memory1 : Memory  InheritSampleTime=on
  Relais ansteuern1 : MATLAB Function  TreatAsAtomicUnit=on
  Sum : Sum  Inputs=|++
  Unterscheidung Blei Gel Roboter an der virtuellen Ladestation : MATLAB Function  TreatAsAtomicUnit=on
  SOC : Outport
  Output_Flag : Outport  Port=2
  wires:
  Relais ansteuern1/1(SOC) -> SOC/1
  Compare To Zero1/1 -> Charging Counter/2
  Gain1/1 -> Data Type Conversion2/1
  Data Type Conversion2/1 -> Relais ansteuern1/2(SOC1)
  Gain/1 -> Data Type Conversion1/1
  Data Type Conversion1/1 -> Relais ansteuern1/3(SOC2)
  Data Type Conversion3/1 -> Relais ansteuern1/1(Laden)
  Compare To Zero/1 -> MATLAB Function1/2(Inc)
  MATLAB Function/1(y) -> Charging Counter/1
  MATLAB Function1/1(y) -> Discharging Counter/1
  Unterscheidung Blei Gel Roboter an der virtuellen Ladestation/1(Laden) -> Data Type Conversion3/1, MATLAB Function/2(Inc), Discharging Counter/2, Compare To Zero/1, Compare To Zero1/1
  Charging Counter/1 -> Memory/1, Gain1/1
  Discharging Counter/1 -> Memory1/1, Sum/1
  Memory/1 -> MATLAB Function/1(Cnt)
  Memory1/1 -> MATLAB Function1/1(Cnt)
  Sum/1 -> Gain/1
  Constant2/1 -> Sum/2
  Input_Flag/1 -> Flag Communication Simulation/1(Input_Flag), Unterscheidung Blei Gel Roboter an der virtuellen Ladestation/1(Input_Flag)
  Flag Communication Simulation/1(Output_Flag) -> Output_Flag/1

== matlab function KitGewerk2_v1_2_Kommunikation_robi/Robotino/transmit velocity, unit & direction converter ==
  settings: sampleTime=2*dtpc
  data: direction_motor0_out output; velocity_motor0_out output; direction_motor1_out output; velocity_motor1_out output; direction_motor2_out output; velocity_motor2_out output; v_x_in input; v_y_in input; v_theta_in input
%%%%%%%%%%%%%%%%%%%%%%%%%%%%%%%%%%%%%%%%%%%%%%%%%%%%%%%%%%%%%%%%%%%%%%%%%%%
% conversion from positive and/or negative longitudinal, lateral and      %
% rotational velocities (in milimeters per second) to three separate      %
% positive motor velocities (resolution: 1Byte) and their rotation        %
% direction                                                               %
%                                                                         %
% inputs:  v_x_in (longitudinal velocity in milimeters per second),       %
%          v_y_in (lateral velocity in milimeters per second),            %
%          v_theta_in (rotational velocity in milimeters per second)      %
% outputs: direction_motor0_out (rotating direction of motor0             %
%          (0 := counter-clockwise; 2 := clockwise)),                     %
%          velocity_motor0_out (from 0 to 255),                           %
%          direction_motor1_out (rotating direction of motor1             %
%          (0 := counter-clockwise; 2 := clockwise)),                     %
%          velocity_motor1_out (from 0 to 255),                           %
%          direction_motor2_out (rotating direction of motor2             %
%          (0 := counter-clockwise; 2 := clockwise)),                     %
%          velocity_motor2_out (from 0 to 255)                            %
%%%%%%%%%%%%%%%%%%%%%%%%%%%%%%%%%%%%%%%%%%%%%%%%%%%%%%%%%%%%%%%%%%%%%%%%%%%
function [direction_motor0_out, velocity_motor0_out, ...
          direction_motor1_out, velocity_motor1_out, ...
          direction_motor2_out, velocity_motor2_out] ...
                                          = fcn(v_x_in, v_y_in, v_theta_in)
%%%%%%%%%%%%%%%%%%%%%%%%%%%%%%%%%%%%%%%%%%%%%%%%%%%%%%%%%%%%%%%%%%%%%%
% conversion from longitudinal, lateral & rotational velocity to the %
% three separate motor velocities                                    %
%%%%%%%%%%%%%%%%%%%%%%%%%%%%%%%%%%%%%%%%%%%%%%%%%%%%%%%%%%%%%%%%%%%%%%
v0 = (-v_x_in * cosd(30)) + ( v_y_in * cosd(60)) + (v_theta_in * 135);
v1 =                      + (-v_y_in)            + (v_theta_in * 135);
v2 = ( v_x_in * cosd(30)) + ( v_y_in * cosd(60)) + (v_theta_in * 135);

%%%%%%%%%%%%%%%%%%%%%%%%%%%%%%%%%%%%%%%%%%%%%%%%%%%%%%%%%%%%%%%%%%%%%
% conversion of the separate motor velocities from millimeters to a %
% value between -255 and 255                                        %
%%%%%%%%%%%%%%%%%%%%%%%%%%%%%%%%%%%%%%%%%%%%%%%%%%%%%%%%%%%%%%%%%%%%%
f = 1 / 7.02;
v0 = v0 * f;
v1 = v1 * f;
v2 = v2 * f;

%%%%%%%%%%%%%%%%%%%%%%%%%%%%%%%%%%%%%%%%%%%%%%%%%%%%%%%%%%%%%%%%%%%%
% division of motor velocities into absolute velocity and rotating %
% direction                                                        %
%%%%%%%%%%%%%%%%%%%%%%%%%%%%%%%%%%%%%%%%%%%%%%%%%%%%%%%%%%%%%%%%%%%%
if v0 < 0
    direction_motor0_out =  0;
    velocity_motor0_out  = -v0;
else
    direction_motor0_out = 2;
    velocity_motor0_out  = v0;
end

if v1 < 0
    direction_motor1_out =  0;
    velocity_motor1_out  = -v1;
else
    direction_motor1_out = 2;
    velocity_motor1_out  = v1;
end

if v2 < 0
    direction_motor2_out =  0;
    velocity_motor2_out  = -v2;
else
    direction_motor2_out = 2;
    velocity_motor2_out  = v2;
end

== matlab function KitGewerk2_v1_2_Kommunikation_robi/Robotino/serial communication/protocol adder & optional velocity adaption ==
  settings: sampleTime=2*dtpc
  data: dir input; vel input; direction_motor0_in input; velocity_motor0_in input; direction_motor1_in input; velocity_motor1_in input; direction_motor2_in input; velocity_motor2_in input; stop_in input; message output
%%%%%%%%%%%%%%%%%%%%%%%%%%%%%%%%%%%%%%%%%%%%%%%%%%%%%%%%%%%%%%%%%%%%%%%%%%%
% parameterising the 'PC104 to I/O-Board message' for serial line         %
% communication with control commands for the robotino motors             %
%                                                                         %
% optional: velocity adaption as soon as at least one motor is near the   %
%           speed limit                                                   %
%                                                                         %
% inputs: rotating directions and velocities of the three motors          %
% output: vector containing the 'PC104 to I/O-Board message' for serial   %
%         line communication                                              %
%%%%%%%%%%%%%%%%%%%%%%%%%%%%%%%%%%%%%%%%%%%%%%%%%%%%%%%%%%%%%%%%%%%%%%%%%%%
function message = fcn(dir, vel, direction_motor0_in, velocity_motor0_in, ...
                       direction_motor1_in, velocity_motor1_in, ...
                       direction_motor2_in, velocity_motor2_in, stop_in)
%%%%%%%%%%%%%%%%%%%%%%%%%%%%%%
% optional velocity adaption %
%%%%%%%%%%%%%%%%%%%%%%%%%%%%%%
vmax = 175;                                               % v_motor_dez_max

if velocity_motor0_in > vmax
    velocity_motor0_tf = velocity_motor0_in;
    
    velocity_motor0_in = vmax;
    velocity_motor1_in = vmax * velocity_motor1_in / velocity_motor0_tf;
    velocity_motor2_in = vmax * velocity_motor2_in / velocity_motor0_tf;
end

if velocity_motor1_in > vmax
    velocity_motor1_tf = velocity_motor1_in;
    
    velocity_motor0_in = vmax * velocity_motor0_in / velocity_motor1_tf;
    velocity_motor1_in = vmax;
    velocity_motor2_in = vmax * velocity_motor2_in / velocity_motor1_tf;
end

if velocity_motor2_in > vmax
    velocity_motor2_tf = velocity_motor2_in;
    
    velocity_motor0_in = vmax * velocity_motor0_in / velocity_motor2_tf;
    velocity_motor1_in = vmax * velocity_motor1_in / velocity_motor2_tf;
    velocity_motor2_in = vmax;
end
%%%%%%%%%%%%%%%%%%%%%%%%%%%%%%%%%%%%%%%%%%%%%%%%%%%%%%%%%%%%%%%%%%%%%%
% vector containing the 'PC104 to I/O-Board message' for serial line %
% communication                                                      %
%%%%%%%%%%%%%%%%%%%%%%%%%%%%%%%%%%%%%%%%%%%%%%%%%%%%%%%%%%%%%%%%%%%%%%
message = [47, abs('REC'), 5, min(stop_in), direction_motor0_in, ...
           velocity_motor0_in, zeros(1, 4), 255, 255, 255, ...
           min(stop_in), direction_motor1_in, velocity_motor1_in, ...
           zeros(1, 4), 255, 255, 255, min(stop_in), ...
           direction_motor2_in, velocity_motor2_in, zeros(1, 4), 255, ...
           255, 255, 1, dir, vel, zeros(1, 4), 255, 255, 255, abs('rec')].';

== matlab function KitGewerk2_v1_2_Kommunikation_robi/UDP interface/stop signals ==
  data: rob_number input; udp_in input; enable_out output
%%%%%%%%%%%%%%%%%%%%%%%%%%%%%%%%%%%%%%%%%%%%%%%%%%%%%%%%%%%%%%%%%%%%%%%%%%%
% Leads the enable command through. The enable command turns the Robotino %
% inputs to selectable form.                                              %
%                                                                         %
% input: udp_in (vector of 56 elements containing the data sent by the    %
%                camera-model)                                            %
% outputs: enable_out (1 = inputs are in selectable form;                 %
%                      0 = inputs are set to 0)                           %
%          udp_out (vector of 56 elements containing the data sent by the %
%                   camera-model)                                         %
%%%%%%%%%%%%%%%%%%%%%%%%%%%%%%%%%%%%%%%%%%%%%%%%%%%%%%%%%%%%%%%%%%%%%%%%%%%
function enable_out  = fcn(rob_number, udp_in)
enable_out = [0, 0];
if (udp_in(rob_number * 3 - 2) <= 0) && ...
   (udp_in(rob_number * 3 - 1) <= 0) && (udp_in(rob_number * 3) <= 0)
    enable_out(1) = 0;
else
    enable_out(1) = 1;
end
enable_out(2) = udp_in(28);
